simulink model "zadanie6"  (R2020a)
settings: Solver=VariableStepAuto  StartTime=0.0  StopTime=10.0  RelTol=1e-3
values from neighbouring files (symbols this model uses):
  K = lqr(sys,Q,R)    [zad6.m]
settings Model: Creator=admin  LastModifiedBy=admin

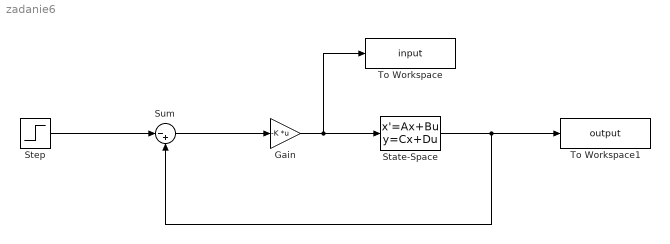
== system zadanie6 ==
  Gain : Gain  Gain=-K  Multiplication=Matrix(K*u)
  State-Space : StateSpace  InitialCondition=0
  Step : Step  SampleTime=0
  Sum : Sum  Inputs=|-+
  To Workspace : ToWorkspace  VariableName=input  SaveFormat=Timeseries  SampleTime=-1
  To Workspace1 : ToWorkspace  VariableName=output  SaveFormat=Timeseries  SampleTime=-1
  wires:
  Step/1 -> Sum/1
  Sum/1 -> Gain/1
  Gain/1 -> To Workspace/1, State-Space/1
  State-Space/1 -> Sum/2, To Workspace1/1
